simulink model "testing_platform_continuous_reaction_cloop_scaled"  (Simulink 7.9)
settings: Solver=ode3  StartTime=0.0  StopTime=1000  FixedStep=ts  MaxStep=100  RelTol=1e-4
values from neighbouring files (symbols this model uses):
  coeff = block.DialogPrm(1).Data    [continuous_reaction_model.m]    (also in continuous_reaction_model_scaled.m; continuous_reaction_model_scaled_sensitivity.m)
  x0 = block.DialogPrm(2).Data    [continuous_reaction_model.m]    (also in continuous_reaction_model_scaled.m; continuous_reaction_model_scaled_sensitivity.m)
undefined symbols (not defined in the file or in its folder): Fss, ts
libraries: cstblocks x1
settings Model: Creator=mforgione  LastModifiedBy=marco
settings OptimizationCC: InitFltsAndDblsToZero=on  AccelVerboseBuild=on
settings DebuggingCC: FcnCallInpInsideContextMsg=Use local settings  StrictBusMsg=Warning
settings GRTTargetCC: CombineOutputUpdateFcns=off  GRTInterface=on

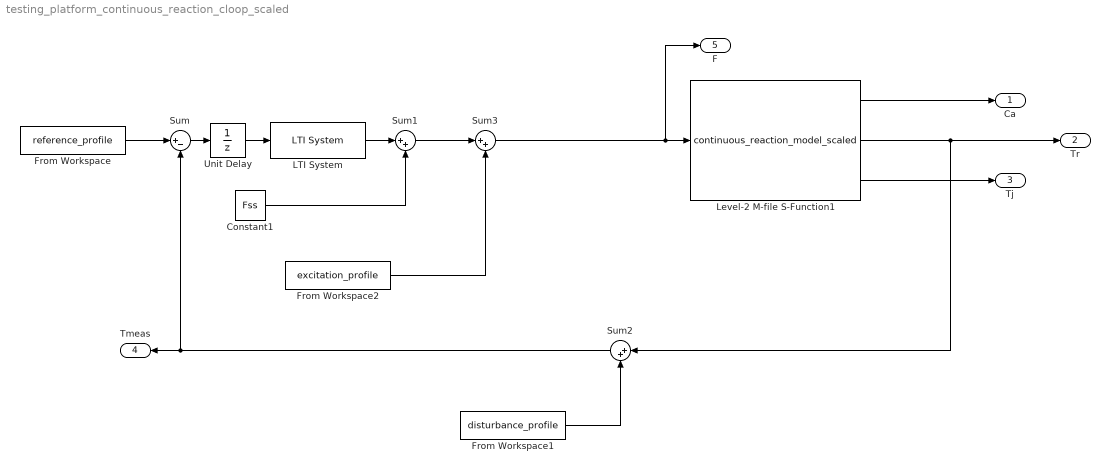
== system testing_platform_continuous_reaction_cloop_scaled ==
  Constant1 : Constant  Value=Fss
  From Workspace : FromWorkspace  VariableName=reference_profile  SampleTime=0
  From Workspace1 : FromWorkspace  VariableName=disturbance_profile  SampleTime=0
  From Workspace2 : FromWorkspace  VariableName=excitation_profile  SampleTime=0
  LTI System : cstblocks/LTI System  sys=C  IC=[]
  Level-2 M-file S-Function1 : M-S-Function  FunctionName=continuous_reaction_model_scaled  Parameters=coeff x0
  Sum : Sum  Inputs=|+-
  Sum1 : Sum  Inputs=|++
  Sum2 : Sum  Inputs=|++
  Sum3 : Sum  Inputs=|++
  Unit Delay : UnitDelay  SampleTime=ts
  Ca : Outport
  Tr : Outport  Port=2
  Tj : Outport  Port=3
  Tmeas : Outport  Port=4
  F : Outport  Port=5
  wires:
  Level-2 M-file S-Function1/1 -> Ca/1
  Level-2 M-file S-Function1/2 -> Tr/1, Sum2/1
  Level-2 M-file S-Function1/3 -> Tj/1
  Sum/1 -> Unit Delay/1
  Constant1/1 -> Sum1/2
  Sum2/1 -> Sum/2, Tmeas/1
  Sum1/1 -> Sum3/1
  Sum3/1 -> Level-2 M-file S-Function1/1, F/1
  LTI System/1 -> Sum1/1
  Unit Delay/1 -> LTI System/1
  From Workspace/1 -> Sum/1
  From Workspace1/1 -> Sum2/2
  From Workspace2/1 -> Sum3/2
